simulink model "IDP2_Shehab_Electrical_Systems_Model"  (R2025b)
settings: Solver=VariableStepAuto  StartTime=0.0  StopTime=20  RelTol=1e-3
libraries: nesl_utility x34, fl_lib x32, ee_lib x21, simulink x6
settings Model: Creator=HP VICTUS  LastModifiedBy=HP VICTUS

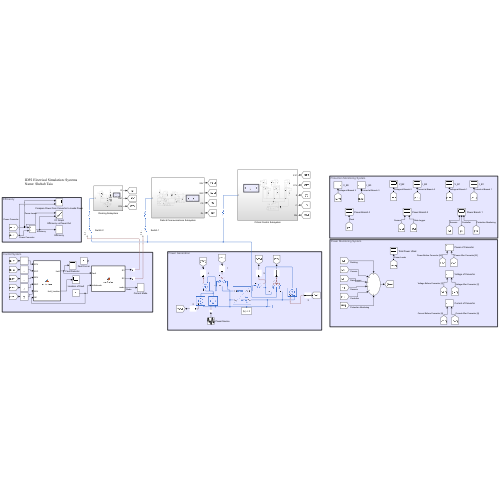
[thumbnail: Simulink's stored preview of the top-level diagram]
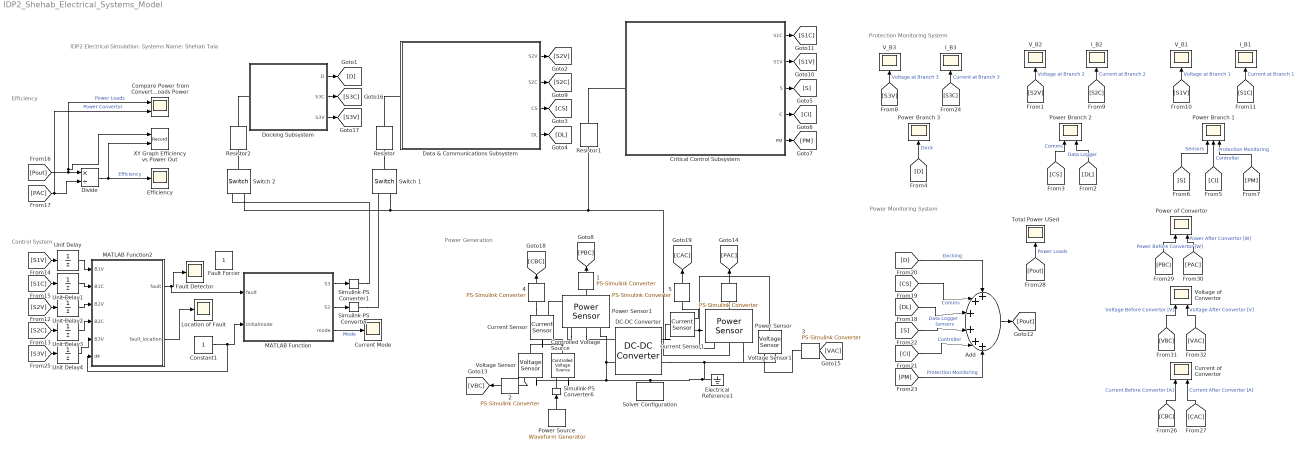
== system IDP2_Shehab_Electrical_Systems_Model ==
  note: Control System
  note: Power Generation
  note: Protection Monitoring System
  note: Power Monitoring System
  note: Efficiency
  note: IDP2 Electrical Simulation: Systems
      | Name: Shehab Taia
   {,1..5} (6 alike) : nesl_utility/PS-Simulink Converter  PhysicalDomain=network_engine_domain  SubClassName=ps_output  LeftPortType=input  RightPortType=output  PseudoPeriodic=off  Frequencies=[]  VectorFormat=1-D array  Unit=1  AffineConversion=off
  Add : Sum  Inputs=++++++
  Compare Power from Convertor to Loads Power : Scope  NumInputPorts=2
      settings: ActiveDisplayYMinimum=79.650776792266242  ActiveDisplayYMaximum=134.0264612610577  DataLoggingVariableName=ScopeData10
  Constant1 : Constant
  Controlled Voltage Source : fl_lib/Electrical/Electrical Sources/Controlled Voltage Source
  Critical Control Subsystem : Subsystem
  Current Mode : Scope
      settings: ActiveDisplayYMinimum=2  ActiveDisplayYMaximum=4  DataLoggingVariableName=ScopeData9
  Current Sensor : fl_lib/Electrical/Electrical Sensors/Current Sensor
  Current Sensor1 : fl_lib/Electrical/Electrical Sensors/Current Sensor
  Current of Convertor : Scope  NumInputPorts=2
      settings: ActiveDisplayYMinimum=0.36664506797171792  ActiveDisplayYMaximum=17.216687272107844  DataLoggingVariableName=ScopeData16
  DC-DC Converter : ee_lib/Semiconductors & Converters/Converters/DC-DC Converter  Vref_option=ee.enum.converters.voltageref.internal  v_ref=24 V  P_rated=250 W  droop_enabled=true  droop_param=ee.enum.converters.droop.value  droop=0.1 V/A  droop_percent=2  Vref_droop=10 V  reversible=ee.enum.converters.directionality.unidirectional  G_diode=1e-8 1/Ohm  P_fixed=2 W  losses_option=ee.enum.converters.lossesOption.proportionalToSquaredCurrent  eff_rated=80  tableOption=ee.enum.converters.lossTableOptionThermal.currentTemp  i_eff_vec=[-2, -1, 1, 2] A  v_eff_vec=[15, 30, 45] V  eff_vec=[66, 76, 80, 74]  eff_2D_table=[66, 66, 66; 76, 76, 76; 80, 80, 80; 74, 74, 74]  model_dynamics=ee.enum.converters.dynamics.yes  tau=0.002 s  v_ini=24 V  v1_min=25 V  R1=1000 Ohm  R2=1000 Ohm  fault_condition=ee.enum.faults.faultInputCondition.greaterThan  fault_threshold=0.5  T_eff_vec=[280, 300, 320] K  eff_3D_table=repmat([66; 76; 80; 74], 1, 3, 3)  thermal_mass=100 J/K  initial_temperature=298.15 K
      settings: InternalSimscapePortConfiguration="{\"Bottom\":[],\"Left\":[{\"id\":\"p1\",\"label\":\"1+\",\"type\":\"foundation.electrical.electrical\"},{\"id\":\"n1\",\"label\":\"1-\",\"type\":\"foundation.electrical.electrical\"}],\"Right\":[{\"id\":\"p2\",\"label\":\"2+\",\"type\":\"foundation.electrical.electrical\"},{\"id\":\"n2\",\"label\":\"2-\",\"type\":\"foundation.electrical.electrical\"}],\"Top\":[]}"
  Data & Communications Subsystem : Subsystem
  Divide : Product  Inputs=*/
  Docking Subsystem : Subsystem
  Efficiency : Scope
      settings: ActiveDisplayYMinimum=0.97227994080182123  ActiveDisplayYMaximum=0.9793482518533968  DataLoggingVariableName=ScopeData11
  Electrical Reference1 : fl_lib/Electrical/Electrical Elements/Electrical Reference
  Fault Detector : Scope
      settings: ActiveDisplayYMinimum=-1.5392337080670928  ActiveDisplayYMaximum=1.140957573182908  DataLoggingVariableName=ScopeData12
  Fault Forcer : Constant
  I_B1 : Scope
      settings: ActiveDisplayYMinimum=2.3119159885086678  ActiveDisplayYMaximum=3.2126875641151642  DataLoggingVariableName=ScopeData8
  I_B2 : Scope
      settings: ActiveDisplayYMinimum=0.94930828791291022  ActiveDisplayYMaximum=2.6489186671968752  DataLoggingVariableName=ScopeData6
  I_B3 : Scope
      settings: ActiveDisplayYMinimum=-1.2813099491745756  ActiveDisplayYMaximum=11.555789758551514  DataLoggingVariableName=ScopeData2
  Location of Fault : Scope
      settings: ActiveDisplayYMinimum=-1  ActiveDisplayYMaximum=1  DataLoggingVariableName=ScopeData3
  MATLAB Function : MATLAB Function  TreatAsAtomicUnit=on
  MATLAB Function2 : MATLAB Function  TreatAsAtomicUnit=on
  Power Branch 1 : Scope  NumInputPorts=3
      settings: ActiveDisplayYMinimum=14.22765652678723  ActiveDisplayYMaximum=23.288334649201424
  Power Branch 2 : Scope  NumInputPorts=2
      settings: ActiveDisplayYMinimum=3.2562727594337782E-13  ActiveDisplayYMaximum=9.0422696415485483E-13
  Power Branch 3 : Scope
      settings: ActiveDisplayYMinimum=-26.0748239794843  ActiveDisplayYMaximum=235.249408902669  DataLoggingVariableName=ScopeData14
  Power Sensor : ee_lib/Sensors & Transducers/Power Sensor  measurement_type=1  averaging_period=1e-4 s
  Power Sensor1 : ee_lib/Sensors & Transducers/Power Sensor  measurement_type=1  averaging_period=1e-4 s
  Power Source : simulink/Sources/Waveform Generator  OutMin=[]  OutMax=[]  OutDataTypeStr=double  SelectedSignal=1  Signals=48 + sin(1, 0.5, 0)  BlockNames=MultiportSwitch_827ba4d7564a4f2  SampleTime=0.1
  Power of Convertor : Scope  NumInputPorts=2
      settings: ActiveDisplayYMinimum=41.30913702815846  ActiveDisplayYMaximum=522.47808402698706  DataLoggingVariableName=ScopeData17
  Resistor : ee_lib/Passive/Resistor  R=0.2 Ohm  enable_R_tol=ee.enum.toleranceApplication.none  R_tol=5  tol_distribution=ee.enum.toleranceDistribution.uniform  nSigma=4  enable_operating_limits=ee.enum.enable.no  operating_limit_action=ee.enum.passive.reportOpLim.warn  power_rating=1 W  max_working_voltage=100 V  noise_mode=ee.enum.sources.noise.Disabled  Tdevice=25 degC  sample_time=1e-3 s  repeatability=ee.enum.ic.repeatability.notRepeatable  user_seed=0  auto_seed=2438775377  power_derating_T1=70 degC  power_derating_T2=155 degC  operating_temperature_range_vec=[-50, 150] degC  alpha=3.93e-3 1/K  Tmeas=25 degC  thermal_mass=100 J/K  temperature_specify=off  temperature_priority=High  temperature=298.15 K  temperature_nominal_specify=off  temperature_nominal_value=1  temperature_nominal_unit=K
  Resistor1 : ee_lib/Passive/Resistor  R=0.2 Ohm  enable_R_tol=ee.enum.toleranceApplication.none  R_tol=5  tol_distribution=ee.enum.toleranceDistribution.uniform  nSigma=4  enable_operating_limits=ee.enum.enable.no  operating_limit_action=ee.enum.passive.reportOpLim.warn  power_rating=1 W  max_working_voltage=100 V  noise_mode=ee.enum.sources.noise.Disabled  Tdevice=25 degC  sample_time=1e-3 s  repeatability=ee.enum.ic.repeatability.notRepeatable  user_seed=0  auto_seed=325791693  power_derating_T1=70 degC  power_derating_T2=155 degC  operating_temperature_range_vec=[-50, 150] degC  alpha=3.93e-3 1/K  Tmeas=25 degC  thermal_mass=100 J/K  temperature_specify=off  temperature_priority=High  temperature=298.15 K  temperature_nominal_specify=off  temperature_nominal_value=1  temperature_nominal_unit=K
  Resistor2 : ee_lib/Passive/Resistor  R=0.2 Ohm  enable_R_tol=ee.enum.toleranceApplication.none  R_tol=5  tol_distribution=ee.enum.toleranceDistribution.uniform  nSigma=4  enable_operating_limits=ee.enum.enable.no  operating_limit_action=ee.enum.passive.reportOpLim.warn  power_rating=1 W  max_working_voltage=100 V  noise_mode=ee.enum.sources.noise.Disabled  Tdevice=25 degC  sample_time=1e-3 s  repeatability=ee.enum.ic.repeatability.notRepeatable  user_seed=0  auto_seed=3807908384  power_derating_T1=70 degC  power_derating_T2=155 degC  operating_temperature_range_vec=[-50, 150] degC  alpha=3.93e-3 1/K  Tmeas=25 degC  thermal_mass=100 J/K  temperature_specify=off  temperature_priority=High  temperature=298.15 K  temperature_nominal_specify=off  temperature_nominal_value=1  temperature_nominal_unit=K
  Simulink-PS Converter : nesl_utility/Simulink-PS Converter  PhysicalDomain=network_engine_domain  SubClassName=ps_input  LeftPortType=input  RightPortType=output  PseudoPeriodic=off  Frequencies=[]  NoiseDistribution=none  NoiseParameters=[]  Unit=1  AffineConversion=off  FilteringAndDerivatives=provide  SimscapeFilterOrder=1  InputFilterTimeConstant=0.001  UdotUserProvided=0
  Simulink-PS Converter1 : nesl_utility/Simulink-PS Converter  PhysicalDomain=network_engine_domain  SubClassName=ps_input  LeftPortType=input  RightPortType=output  PseudoPeriodic=off  Frequencies=[]  NoiseDistribution=none  NoiseParameters=[]  Unit=1  AffineConversion=off  FilteringAndDerivatives=provide  SimscapeFilterOrder=1  InputFilterTimeConstant=0.001  UdotUserProvided=0
  Simulink-PS Converter6 : nesl_utility/Simulink-PS Converter  PhysicalDomain=network_engine_domain  SubClassName=ps_input  LeftPortType=input  RightPortType=output  PseudoPeriodic=off  Frequencies=[]  NoiseDistribution=none  NoiseParameters=[]  Unit=1  AffineConversion=off  FilteringAndDerivatives=filter  SimscapeFilterOrder=1  InputFilterTimeConstant=0.001  UdotUserProvided=0
  Solver Configuration : nesl_utility/Solver Configuration  PhysicalDomain=network_engine_domain  SubClassName=solver  LeftPortType=input  RightPortType=generic  Tones=[]  Harmonics=[]  SimulateNoise=off  Profile=off  UseLocalSampling=off  EnableSwitchedLinearOptims=on  FrequencyDomain=off  UseCCode=off  RelTol=0.001  AbsTol=1e-06  MinStep=1e-09  ToWorkspace=off  RevertToSquareIcSolve=off  NumHomotopyIterations=100  PhasorMode=off  PhasorModeNumHarmonics=1  ConsistencySolver=NEWTON_FTOL  IndexReductionMethod=DerivativeReplacement  DoDC=off  ResidualTolerance=1e-09  ConsistencyTolSource=GLOBAL  ConsistencyAbsTol=0.001  ConsistencyRelTol=0.001  ConsistencyTolFactor=0.001  UseLocalSolver=off  LocalSolverChoice=NE_BACKWARD_EULER_ADVANCER  ResolveIndetEquations=on  FunctionEvalNumThread=1  LocalSolverSampleTime=0.001  DoFixedCost=off  MaxNonlinIter=3  MaxModeIter=2  ComputeImpulses=off  ImpulseIterations=2  LinearAlgebra=Sparse  LinearAlgebraNumThread=0  EquationFormulation=NE_TIME_EF  DelaysMemoryBudget=1024  AutomaticFiltering=on  FilteringTimeConstant=0.001  PartitionStorageMethod=AS_NEEDED  PartitionMemoryBudget=1024  PartitionMethod=FAST  MultibodyUseLocalSolver=off  MultibodyLocalSolverChoice=ODE1  MultibodyLocalSolverSampleTime=0.001
  Switch 1 : fl_lib/Electrical/Electrical Elements/Switch  R_closed=0.01 Ohm  G_open=1e-8 1/Ohm  Threshold=0.5  i_specify=off  i_priority=None  i=0 A  i_nominal_specify=off  i_nominal_value=1  i_nominal_unit=A  v_specify=off  v_priority=None  v=0 V  v_nominal_specify=off  v_nominal_value=1  v_nominal_unit=V
  Switch 2 : fl_lib/Electrical/Electrical Elements/Switch  R_closed=0.01 Ohm  G_open=1e-8 1/Ohm  Threshold=0.5  i_specify=off  i_priority=None  i=0 A  i_nominal_specify=off  i_nominal_value=1  i_nominal_unit=A  v_specify=off  v_priority=None  v=0 V  v_nominal_specify=off  v_nominal_value=1  v_nominal_unit=V
  Total Power USed : Scope
      settings: ActiveDisplayYMinimum=57.08705193849255  ActiveDisplayYMaximum=75.545974460086583  DataLoggingVariableName=ScopeData23
  Unit Delay{,1..4} (5 alike) : UnitDelay  InitialCondition=23  SampleTime=-1  HasFrameUpgradeWarning=on
  V_B1 : Scope
      settings: ActiveDisplayYMinimum=21.641364909946656  ActiveDisplayYMaximum=23.691224490128249  DataLoggingVariableName=ScopeData7
  V_B2 : Scope
      settings: ActiveDisplayYMinimum=21.473361802637658  ActiveDisplayYMaximum=24.098708881242768  DataLoggingVariableName=ScopeData5
  V_B3 : Scope
      settings: ActiveDisplayYMinimum=-0.000306600792252615  ActiveDisplayYMaximum=0.0027003867944249715  DataLoggingVariableName=ScopeData4
  Voltage Sensor : fl_lib/Electrical/Electrical Sensors/Voltage Sensor
  Voltage Sensor1 : fl_lib/Electrical/Electrical Sensors/Voltage Sensor
  Voltage of Convertor : Scope  NumInputPorts=2
      settings: ActiveDisplayYMinimum=19.1344610769676  ActiveDisplayYMaximum=52.318383780373431  DataLoggingVariableName=ScopeData18
  XY Graph Efficiency vs Power Out : Record  NumPorts=2.0  FileSettingsInternal="{\"entries\":[{\"content\":{\"excelSettings\":{\"content\":{},\"type\":\"Streamout.ExcelSettings\"},\"parquetSettings\":{\"content\":{},\"type\":\"Streamout.ParquetSettings\"}},\"type\":\"Streamout.FileSettingStorage\",\"uuid\":\"\"}],\"packageUris\":[\"http:\\/\\/schema.mathworks.com\\/mf0\\/streamout_blocks\\/R2020a\"],\"version\":\"1.0\"}"  FrameSettings=[0, 0]  Layout=[1 1]  SignalsInternal="{\"entries\":[{\"content\":{\"signals\":[{\"content\":{\"blockPath\":[],\"dimensions\":[1],\"domain\":\"\",\"lineColor\":\"#a2142f\",\"plots\":[ 1 ],\"port\":1,\"signalID\":1,\"signalName\":\"Power Loads\"},\"type\":\"RecordBlkView.Signal\",\"uuid\":\"\"},{\"content\":{\"blockPath\":[],\"dimensions\":[1],\"domain\":\"\",\"lineColor\":\"#139fff\",\"plots\":[ 1 ],\"port\":2,\"signalID\":2,\"signalName\":\"Efficiency\"},\"type\":\"RecordBlkView.Signal\",\"uuid\":\"\"}]},\"type\":\"RecordBlkView.InputSignals\",\"uuid\":\"\"}],\"packageUris\":[\"http:\\/\\/schema.mathworks.com\\/mf0\\/streamout_blocks\\/R2020a\"],\"version\":\"1.0\"}"  VisualizationBindings="{\"xyplotplugin\":{\"info\":[{\"series\":[{\"bindingParametersList\":[{\"parameter\":\"X-Axis\",\"signalID\":1,\"signalName\":\"Power Loads\"},{\"parameter\":\"Y-Axis\",\"signalID\":2,\"signalName\":\"Efficiency\"}],\"seriesID\":0}],\"subplotID\":1}]}}"  CompatibilityTag=XY  st=-1
  wires:
  Divide/1 -> XY Graph Efficiency vs Power Out/2, Efficiency/1  "Efficiency"
  [Pout] -> Compare Power from Convertor to Loads Power/1, XY Graph Efficiency vs Power Out/1, Divide/1  "Power Loads"
  [PAC] -> Divide/2, Compare Power from Convertor to Loads Power/2  "Power Convertor"
  MATLAB Function2/2(fault_location) -> Location of Fault/1
  " "/1 -> [PAC]
  Power Source/1 -> Simulink-PS Converter6/1
  Docking Subsystem/1(D) -> [D]
  Data & Communications Subsystem/1(S2V) -> [S2V]
  Data & Communications Subsystem/2(S2C) -> [S2C]
  Data & Communications Subsystem/3(CS) -> [CS]
  Data & Communications Subsystem/4(DL) -> [DL]
  Critical Control Subsystem/1(S1C) -> [S1C]
  Critical Control Subsystem/2(S1V) -> [S1V]
  Critical Control Subsystem/3(S) -> [S]
  Critical Control Subsystem/4(C) -> [CI]
  Critical Control Subsystem/5(PM) -> [PM]
  MATLAB Function/2(S2) -> Simulink-PS Converter/1
  MATLAB Function/1(S3) -> Simulink-PS Converter1/1
  MATLAB Function/3(mode) -> Current Mode/1  "Mode"
  [S2V] -> V_B2/1  "Voltage at Branch 2"
  [S2C] -> I_B2/1  "Current at Branch 2"
  [S1V] -> V_B1/1  "Voltage at Branch 1"
  [S1C] -> I_B1/1  "Current at Branch 1"
  [CS] -> Power Branch 2/1  "Comms"
  [DL] -> Power Branch 2/2  "Data Logger"
  [S] -> Power Branch 1/1  "Sensors"
  [CI] -> Power Branch 1/2  "Controller"
  [PM] -> Power Branch 1/3  "Protection Monitoring"
  [VAC] -> Voltage of Convertor/2  "Voltage After Convertor [V]"
  [VBC] -> Voltage of Convertor/1  "Voltage Before Convertor [V]"
  [PBC] -> Power of Convertor/1  "Power Before Convertor [W]"
  [D] -> Add/1  "Docking"
  [CS] -> Add/2  "Comms"
  [DL] -> Add/3  "Data Logger"
  [S] -> Add/4  "Sensors"
  [CI] -> Add/5  "Controller"
  [PM] -> Add/6  "Protection Monitoring"
  Add/1 -> [Pout]
  " 3"/1 -> [VAC]
  [PAC] -> Power of Convertor/2  "Power After Convertor [W]"
  " 2"/1 -> [VBC]
  Docking Subsystem/2(S3C) -> [S3C]
  Docking Subsystem/3(S3V) -> [S3V]
  [S3C] -> I_B3/1  "Current at Branch 3"
  [S3V] -> V_B3/1  "Voltage at Branch 3"
  [S1V] -> Unit Delay/1
  [S2C] -> Unit Delay3/1
  [S1C] -> Unit Delay1/1
  [S2V] -> Unit Delay2/1
  [S3V] -> Unit Delay4/1
  Unit Delay3/1 -> MATLAB Function2/4(B2C)
  Unit Delay2/1 -> MATLAB Function2/3(B2V)
  Unit Delay1/1 -> MATLAB Function2/2(B1C)
  Unit Delay/1 -> MATLAB Function2/1(B1V)
  Unit Delay4/1 -> MATLAB Function2/5(B3V)
  Constant1/1 -> MATLAB Function2/6(IM), MATLAB Function/2(initialmode)
  MATLAB Function2/1(fault) -> MATLAB Function/1(fault), Fault Detector/1
  " 4"/1 -> [CBC]
  " 5"/1 -> [CAC]
  [CBC] -> Current of Convertor/1  "Current Before Convertor [A]"
  [CAC] -> Current of Convertor/2  "Current After Convertor [A]"
  " 1"/1 -> [PBC]
  [D] -> Power Branch 3/1  "Dock"
  [Pout] -> Total Power USed/1  "Power Loads"
  connections:
  Power Sensor1/LConn1 -- Current Sensor/RConn2
  Simulink-PS Converter6/RConn1 -- Controlled Voltage Source/RConn1
  Resistor/LConn1 -- Switch 1/LConn1
  Switch 1/RConn2 -- Power Sensor/LConn2 -- Resistor1/LConn1 -- Switch 2/RConn2
  Switch 2/LConn1 -- Resistor2/LConn1
  Resistor/RConn1 -- Data & Communications Subsystem/LConn1
  DC-DC Converter/RConn2 -- Power Sensor/LConn3 -- Voltage Sensor1/RConn2 -- Solver Configuration/RConn1 -- Voltage Sensor/RConn2 -- Controlled Voltage Source/RConn2 -- Power Sensor1/LConn3 -- DC-DC Converter/LConn2 -- Electrical Reference1/LConn1
  Critical Control Subsystem/LConn1 -- Resistor1/RConn1
  Voltage Sensor1/LConn1 -- Power Sensor/LConn1 -- Current Sensor1/RConn2
  " "/LConn1 -- Power Sensor/RConn1
  Power Sensor1/RConn1 -- " 1"/LConn1
  " 2"/LConn1 -- Voltage Sensor/RConn1
  " 3"/LConn1 -- Voltage Sensor1/RConn1
  Power Sensor1/LConn2 -- DC-DC Converter/LConn1
  Simulink-PS Converter1/RConn1 -- Switch 2/RConn1
  Simulink-PS Converter/RConn1 -- Switch 1/RConn1
  Resistor2/RConn1 -- Docking Subsystem/LConn1
  Current Sensor/LConn1 -- Controlled Voltage Source/LConn1 -- Voltage Sensor/LConn1
  " 4"/LConn1 -- Current Sensor/RConn1
  DC-DC Converter/RConn1 -- Current Sensor1/LConn1
  " 5"/LConn1 -- Current Sensor1/RConn1

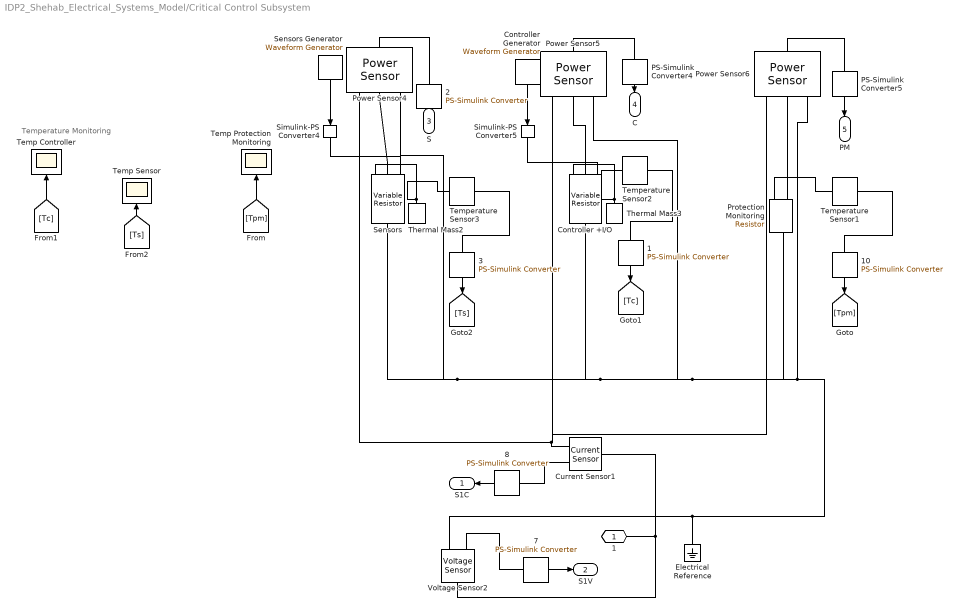
== system IDP2_Shehab_Electrical_Systems_Model/Critical Control Subsystem ==
  note: Temperature Monitoring
   {1..3,7..8,10} (6 alike) : nesl_utility/PS-Simulink Converter  PhysicalDomain=network_engine_domain  SubClassName=ps_output  LeftPortType=input  RightPortType=output  PseudoPeriodic=off  Frequencies=[]  VectorFormat=1-D array  Unit=1  AffineConversion=off
  Controller Generator : simulink/Sources/Waveform Generator  OutMin=[]  OutMax=[]  OutDataTypeStr=double  SelectedSignal=1  Signals=step(5, 23.04, 16.46) + step(6, 0, 6.58)  BlockNames=MultiportSwitch_3dca4f294659435  SampleTime=0.1
  Controller +I/O : fl_lib/Electrical/Electrical Elements/Variable Resistor  Rmin=0 Ohm  thermalEnable=true  thermal_mass=0 J/K  i_specify=off  i_priority=None  i=0 A  i_nominal_specify=off  i_nominal_value=1  i_nominal_unit=A  v_specify=off  v_priority=None  v=0 V  v_nominal_specify=off  v_nominal_value=1  v_nominal_unit=V  T_specify=off  T_priority=None  T=300 K  T_nominal_specify=off  T_nominal_value=1  T_nominal_unit=K
      settings: InternalSimscapePortConfiguration="{\"Bottom\":[],\"Left\":[{\"id\":\"R\",\"label\":\"R\",\"type\":\"input\"},{\"id\":\"p\",\"label\":\"+\",\"type\":\"foundation.electrical.electrical\"}],\"Right\":[{\"id\":\"n\",\"label\":\"-\",\"type\":\"foundation.electrical.electrical\"}],\"Top\":[{\"id\":\"H\",\"label\":\"H\",\"type\":\"foundation.thermal.thermal\"}]}"
  Current Sensor1 : fl_lib/Electrical/Electrical Sensors/Current Sensor
  Electrical Reference : fl_lib/Electrical/Electrical Elements/Electrical Reference
  PS-Simulink Converter4 : nesl_utility/PS-Simulink Converter  PhysicalDomain=network_engine_domain  SubClassName=ps_output  LeftPortType=input  RightPortType=output  PseudoPeriodic=off  Frequencies=[]  VectorFormat=1-D array  Unit=1  AffineConversion=off
  PS-Simulink Converter5 : nesl_utility/PS-Simulink Converter  PhysicalDomain=network_engine_domain  SubClassName=ps_output  LeftPortType=input  RightPortType=output  PseudoPeriodic=off  Frequencies=[]  VectorFormat=1-D array  Unit=1  AffineConversion=off
  Power Sensor4 : ee_lib/Sensors & Transducers/Power Sensor  measurement_type=1  averaging_period=1e-4 s
  Power Sensor5 : ee_lib/Sensors & Transducers/Power Sensor  measurement_type=1  averaging_period=1e-4 s
  Power Sensor6 : ee_lib/Sensors & Transducers/Power Sensor  measurement_type=1  averaging_period=1e-4 s
  Protection Monitoring : ee_lib/Passive/Resistor  R=28.8 Ohm  enable_R_tol=ee.enum.toleranceApplication.none  R_tol=5  tol_distribution=ee.enum.toleranceDistribution.uniform  nSigma=4  enable_operating_limits=ee.enum.enable.no  operating_limit_action=ee.enum.passive.reportOpLim.warn  power_rating=1 W  max_working_voltage=100 V  noise_mode=ee.enum.sources.noise.Disabled  Tdevice=25 degC  sample_time=1e-3 s  repeatability=ee.enum.ic.repeatability.notRepeatable  user_seed=0  auto_seed=1119815447  power_derating_T1=70 degC  power_derating_T2=155 degC  operating_temperature_range_vec=[-50, 150] degC  alpha=3.93e-3 1/K  Tmeas=25 degC  thermal_mass=200 J/K  temperature_specify=off  temperature_priority=High  temperature=298.15 K  temperature_nominal_specify=off  temperature_nominal_value=1  temperature_nominal_unit=K
      settings: InternalSimscapePortConfiguration="{\"Bottom\":[],\"Left\":[{\"id\":\"p\",\"label\":\"+\",\"type\":\"foundation.electrical.electrical\"},{\"id\":\"H\",\"label\":\"H\",\"type\":\"foundation.thermal.thermal\"}],\"Right\":[{\"id\":\"n\",\"label\":\"-\",\"type\":\"foundation.electrical.electrical\"}],\"Top\":[]}"
  Sensors : fl_lib/Electrical/Electrical Elements/Variable Resistor  Rmin=0 Ohm  thermalEnable=true  thermal_mass=0 J/K  i_specify=off  i_priority=None  i=0 A  i_nominal_specify=off  i_nominal_value=1  i_nominal_unit=A  v_specify=off  v_priority=None  v=0 V  v_nominal_specify=off  v_nominal_value=1  v_nominal_unit=V  T_specify=off  T_priority=None  T=300 K  T_nominal_specify=off  T_nominal_value=1  T_nominal_unit=K
      settings: InternalSimscapePortConfiguration="{\"Bottom\":[],\"Left\":[{\"id\":\"R\",\"label\":\"R\",\"type\":\"input\"},{\"id\":\"p\",\"label\":\"+\",\"type\":\"foundation.electrical.electrical\"}],\"Right\":[{\"id\":\"n\",\"label\":\"-\",\"type\":\"foundation.electrical.electrical\"}],\"Top\":[{\"id\":\"H\",\"label\":\"H\",\"type\":\"foundation.thermal.thermal\"}]}"
  Sensors Generator : simulink/Sources/Waveform Generator  OutMin=[]  OutMax=[]  OutDataTypeStr=double  SelectedSignal=1  Signals=step(3, 32, 23.04) + step(10, 0, 32-23.04)  BlockNames=MultiportSwitch_565f76e57e2d47f  SampleTime=0.1
  Simulink-PS Converter4 : nesl_utility/Simulink-PS Converter  PhysicalDomain=network_engine_domain  SubClassName=ps_input  LeftPortType=input  RightPortType=output  PseudoPeriodic=off  Frequencies=[]  NoiseDistribution=none  NoiseParameters=[]  Unit=1  AffineConversion=off  FilteringAndDerivatives=filter  SimscapeFilterOrder=1  InputFilterTimeConstant=0.001  UdotUserProvided=0
  Simulink-PS Converter5 : nesl_utility/Simulink-PS Converter  PhysicalDomain=network_engine_domain  SubClassName=ps_input  LeftPortType=input  RightPortType=output  PseudoPeriodic=off  Frequencies=[]  NoiseDistribution=none  NoiseParameters=[]  Unit=1  AffineConversion=off  FilteringAndDerivatives=filter  SimscapeFilterOrder=1  InputFilterTimeConstant=0.001  UdotUserProvided=0
  Temp Controller : Scope
      settings: ActiveDisplayYMinimum=292.94814557194843  ActiveDisplayYMaximum=294.96668985246413  DataLoggingVariableName=ScopeData19
  Temp Protection Monitoring : Scope
      settings: ActiveDisplayYMinimum=297.9369765879818  ActiveDisplayYMaximum=300.06721070816349  DataLoggingVariableName=ScopeData13
  Temp Sensor : Scope
      settings: ActiveDisplayYMinimum=292.66432897393719  ActiveDisplayYMaximum=297.52103923456542  DataLoggingVariableName=ScopeData20
  Temperature Sensor1 : fl_lib/Thermal/Thermal Sensors/Temperature Sensor  temperature_measure=foundation.enum.MeasurementReference.absolute
      settings: InternalSimscapePortConfiguration="{\"Bottom\":[],\"Left\":[{\"id\":\"A\",\"label\":\"A\",\"type\":\"foundation.thermal.thermal\"}],\"Right\":[{\"id\":\"T\",\"label\":\"T\",\"type\":\"output\"}],\"Top\":[]}"
  Temperature Sensor2 : fl_lib/Thermal/Thermal Sensors/Temperature Sensor  temperature_measure=foundation.enum.MeasurementReference.absolute
      settings: InternalSimscapePortConfiguration="{\"Bottom\":[],\"Left\":[{\"id\":\"A\",\"label\":\"A\",\"type\":\"foundation.thermal.thermal\"}],\"Right\":[{\"id\":\"T\",\"label\":\"T\",\"type\":\"output\"}],\"Top\":[]}"
  Temperature Sensor3 : fl_lib/Thermal/Thermal Sensors/Temperature Sensor  temperature_measure=foundation.enum.MeasurementReference.absolute
      settings: InternalSimscapePortConfiguration="{\"Bottom\":[],\"Left\":[{\"id\":\"A\",\"label\":\"A\",\"type\":\"foundation.thermal.thermal\"}],\"Right\":[{\"id\":\"T\",\"label\":\"T\",\"type\":\"output\"}],\"Top\":[]}"
  Thermal Mass2 : fl_lib/Thermal/Thermal Elements/Thermal Mass  mass_type=foundation.enum.constant_variable.constant  mass=1 kg  sp_heat=90 J/(K*kg)  mass_min=1e-6 kg  num_ports=foundation.enum.numPorts2.one  m_specify=off  m_priority=High  m=1 kg  m_nominal_specify=off  m_nominal_value=1  m_nominal_unit=kg  T_specify=on  T_priority=Low  T=293.15 K  T_nominal_specify=off  T_nominal_value=1  T_nominal_unit=K  Q_specify=off  Q_priority=None  Q=0 W  Q_nominal_specify=off  Q_nominal_value=1  Q_nominal_unit=W
  Thermal Mass3 : fl_lib/Thermal/Thermal Elements/Thermal Mass  mass_type=foundation.enum.constant_variable.constant  mass=1 kg  sp_heat=270 J/(K*kg)  mass_min=1e-6 kg  num_ports=foundation.enum.numPorts2.one  m_specify=off  m_priority=High  m=1 kg  m_nominal_specify=off  m_nominal_value=1  m_nominal_unit=kg  T_specify=on  T_priority=Low  T=293.15 K  T_nominal_specify=off  T_nominal_value=1  T_nominal_unit=K  Q_specify=off  Q_priority=None  Q=0 W  Q_nominal_specify=off  Q_nominal_value=1  Q_nominal_unit=W
  Voltage Sensor2 : fl_lib/Electrical/Electrical Sensors/Voltage Sensor
  1 : PMIOPort  Side=Left
  S1C : Outport
  S1V : Outport  Port=2
  S : Outport  Port=3
  C : Outport  Port=4
  PM : Outport  Port=5
  wires:
  Controller Generator/1 -> Simulink-PS Converter5/1
  Sensors Generator/1 -> Simulink-PS Converter4/1
  " 2"/1 -> S/1
  " 8"/1 -> S1C/1
  " 7"/1 -> S1V/1
  PS-Simulink Converter4/1 -> C/1
  PS-Simulink Converter5/1 -> PM/1
  " 10"/1 -> [Tpm]
  [Tpm] -> Temp Protection Monitoring/1
  [Tc] -> Temp Controller/1
  [Ts] -> Temp Sensor/1
  " 1"/1 -> [Tc]
  " 3"/1 -> [Ts]
  connections:
  Power Sensor6/LConn3 -- Protection Monitoring/RConn1 -- Power Sensor5/LConn3 -- Controller +I/O/RConn1 -- Power Sensor4/LConn3 -- Sensors/RConn1 -- Voltage Sensor2/RConn2 -- Electrical Reference/LConn1
  Current Sensor1/RConn1 -- " 8"/LConn1
  Temperature Sensor1/LConn1 -- Protection Monitoring/LConn2
  Power Sensor6/LConn2 -- Protection Monitoring/LConn1
  Thermal Mass3/LConn1 -- Temperature Sensor2/LConn1 -- Controller +I/O/LConn3
  PS-Simulink Converter4/LConn1 -- Power Sensor5/RConn1
  " 10"/LConn1 -- Temperature Sensor1/RConn1
  Current Sensor1/LConn1 -- Voltage Sensor2/LConn1 -- 1/RConn1
  PS-Simulink Converter5/LConn1 -- Power Sensor6/RConn1
  Thermal Mass2/LConn1 -- Temperature Sensor3/LConn1 -- Sensors/LConn3
  Current Sensor1/RConn2 -- Power Sensor6/LConn1 -- Power Sensor5/LConn1 -- Power Sensor4/LConn1
  Power Sensor5/LConn2 -- Controller +I/O/LConn2
  Controller +I/O/LConn1 -- Simulink-PS Converter5/RConn1
  " 2"/LConn1 -- Power Sensor4/RConn1
  Simulink-PS Converter4/RConn1 -- Sensors/LConn1
  Voltage Sensor2/RConn1 -- " 7"/LConn1
  Sensors/LConn2 -- Power Sensor4/LConn2
  " 1"/LConn1 -- Temperature Sensor2/RConn1
  " 3"/LConn1 -- Temperature Sensor3/RConn1

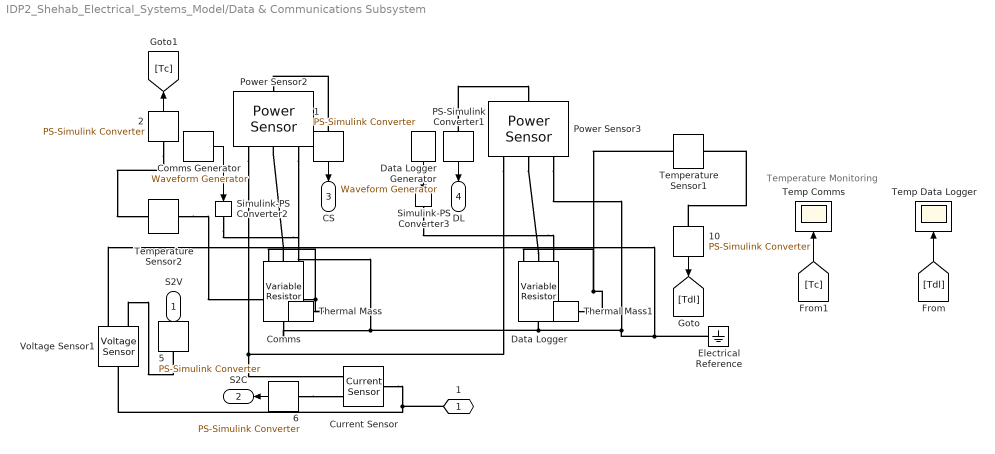
== system IDP2_Shehab_Electrical_Systems_Model/Data & Communications Subsystem ==
  note: Temperature Monitoring
   {1..2,5..6,10} (5 alike) : nesl_utility/PS-Simulink Converter  PhysicalDomain=network_engine_domain  SubClassName=ps_output  LeftPortType=input  RightPortType=output  PseudoPeriodic=off  Frequencies=[]  VectorFormat=1-D array  Unit=1  AffineConversion=off
  Comms : fl_lib/Electrical/Electrical Elements/Variable Resistor  Rmin=0 Ohm  thermalEnable=true  thermal_mass=0 J/K  i_specify=off  i_priority=None  i=0 A  i_nominal_specify=off  i_nominal_value=1  i_nominal_unit=A  v_specify=off  v_priority=None  v=0 V  v_nominal_specify=off  v_nominal_value=1  v_nominal_unit=V  T_specify=off  T_priority=None  T=300 K  T_nominal_specify=off  T_nominal_value=1  T_nominal_unit=K
      settings: InternalSimscapePortConfiguration="{\"Bottom\":[],\"Left\":[{\"id\":\"R\",\"label\":\"R\",\"type\":\"input\"},{\"id\":\"p\",\"label\":\"+\",\"type\":\"foundation.electrical.electrical\"}],\"Right\":[{\"id\":\"n\",\"label\":\"-\",\"type\":\"foundation.electrical.electrical\"}],\"Top\":[{\"id\":\"H\",\"label\":\"H\",\"type\":\"foundation.thermal.thermal\"}]}"
  Comms Generator : simulink/Sources/Waveform Generator  OutMin=[]  OutMax=[]  OutDataTypeStr=double  SelectedSignal=1  Signals=step(5, 28.8, 11.52)  BlockNames=MultiportSwitch_095543f3cf194af  SampleTime=0.1
  Current Sensor : fl_lib/Electrical/Electrical Sensors/Current Sensor
  Data Logger : fl_lib/Electrical/Electrical Elements/Variable Resistor  Rmin=0 Ohm  thermalEnable=true  thermal_mass=0 J/K  i_specify=off  i_priority=None  i=0 A  i_nominal_specify=off  i_nominal_value=1  i_nominal_unit=A  v_specify=off  v_priority=None  v=0 V  v_nominal_specify=off  v_nominal_value=1  v_nominal_unit=V  T_specify=off  T_priority=None  T=300 K  T_nominal_specify=off  T_nominal_value=1  T_nominal_unit=K
      settings: InternalSimscapePortConfiguration="{\"Bottom\":[],\"Left\":[{\"id\":\"R\",\"label\":\"R\",\"type\":\"input\"},{\"id\":\"p\",\"label\":\"+\",\"type\":\"foundation.electrical.electrical\"}],\"Right\":[{\"id\":\"n\",\"label\":\"-\",\"type\":\"foundation.electrical.electrical\"}],\"Top\":[{\"id\":\"H\",\"label\":\"H\",\"type\":\"foundation.thermal.thermal\"}]}"
  Data Logger Generator : simulink/Sources/Waveform Generator  OutMin=[]  OutMax=[]  OutDataTypeStr=double  SelectedSignal=1  Signals=step(7, 72, 38.4)  BlockNames=MultiportSwitch_7b4fce7a58b2408  SampleTime=0.1
  Electrical Reference : fl_lib/Electrical/Electrical Elements/Electrical Reference
  PS-Simulink Converter1 : nesl_utility/PS-Simulink Converter  PhysicalDomain=network_engine_domain  SubClassName=ps_output  LeftPortType=input  RightPortType=output  PseudoPeriodic=off  Frequencies=[]  VectorFormat=1-D array  Unit=1  AffineConversion=off
  Power Sensor2 : ee_lib/Sensors & Transducers/Power Sensor  measurement_type=1  averaging_period=1e-4 s
  Power Sensor3 : ee_lib/Sensors & Transducers/Power Sensor  measurement_type=1  averaging_period=1e-4 s
  Simulink-PS Converter2 : nesl_utility/Simulink-PS Converter  PhysicalDomain=network_engine_domain  SubClassName=ps_input  LeftPortType=input  RightPortType=output  PseudoPeriodic=off  Frequencies=[]  NoiseDistribution=none  NoiseParameters=[]  Unit=1  AffineConversion=off  FilteringAndDerivatives=filter  SimscapeFilterOrder=1  InputFilterTimeConstant=0.001  UdotUserProvided=0
  Simulink-PS Converter3 : nesl_utility/Simulink-PS Converter  PhysicalDomain=network_engine_domain  SubClassName=ps_input  LeftPortType=input  RightPortType=output  PseudoPeriodic=off  Frequencies=[]  NoiseDistribution=none  NoiseParameters=[]  Unit=1  AffineConversion=off  FilteringAndDerivatives=filter  SimscapeFilterOrder=1  InputFilterTimeConstant=0.001  UdotUserProvided=0
  Temp Comms : Scope
      settings: ActiveDisplayYMinimum=292.94814557194843  ActiveDisplayYMaximum=294.96668985246413  DataLoggingVariableName=ScopeData21
  "Temp Data Logger " : Scope
      settings: ActiveDisplayYMinimum=293.00152884444793  ActiveDisplayYMaximum=294.48624039996855  DataLoggingVariableName=ScopeData22
  Temperature Sensor1 : fl_lib/Thermal/Thermal Sensors/Temperature Sensor  temperature_measure=foundation.enum.MeasurementReference.absolute
      settings: InternalSimscapePortConfiguration="{\"Bottom\":[],\"Left\":[{\"id\":\"A\",\"label\":\"A\",\"type\":\"foundation.thermal.thermal\"}],\"Right\":[{\"id\":\"T\",\"label\":\"T\",\"type\":\"output\"}],\"Top\":[]}"
  Temperature Sensor2 : fl_lib/Thermal/Thermal Sensors/Temperature Sensor  temperature_measure=foundation.enum.MeasurementReference.absolute
      settings: InternalSimscapePortConfiguration="{\"Bottom\":[],\"Left\":[{\"id\":\"A\",\"label\":\"A\",\"type\":\"foundation.thermal.thermal\"}],\"Right\":[{\"id\":\"T\",\"label\":\"T\",\"type\":\"output\"}],\"Top\":[]}"
  Thermal Mass : fl_lib/Thermal/Thermal Elements/Thermal Mass  mass_type=foundation.enum.constant_variable.constant  mass=1 kg  sp_heat="500  J/(K*kg)"  mass_min=1e-6 kg  num_ports=foundation.enum.numPorts2.one  m_specify=off  m_priority=High  m=1 kg  m_nominal_specify=off  m_nominal_value=1  m_nominal_unit=kg  T_specify=on  T_priority=Low  T=293.15 K  T_nominal_specify=off  T_nominal_value=1  T_nominal_unit=K  Q_specify=off  Q_priority=None  Q=0 W  Q_nominal_specify=off  Q_nominal_value=1  Q_nominal_unit=W
  Thermal Mass1 : fl_lib/Thermal/Thermal Elements/Thermal Mass  mass_type=foundation.enum.constant_variable.constant  mass=1 kg  sp_heat=180 J/(K*kg)  mass_min=1e-6 kg  num_ports=foundation.enum.numPorts2.one  m_specify=off  m_priority=High  m=1 kg  m_nominal_specify=off  m_nominal_value=1  m_nominal_unit=kg  T_specify=on  T_priority=Low  T=293.15 K  T_nominal_specify=off  T_nominal_value=1  T_nominal_unit=K  Q_specify=off  Q_priority=None  Q=0 W  Q_nominal_specify=off  Q_nominal_value=1  Q_nominal_unit=W
  Voltage Sensor1 : fl_lib/Electrical/Electrical Sensors/Voltage Sensor
  1 : PMIOPort  Side=Left
  S2V : Outport
  S2C : Outport  Port=2
  CS : Outport  Port=3
  DL : Outport  Port=4
  wires:
  Comms Generator/1 -> Simulink-PS Converter2/1
  Data Logger Generator/1 -> Simulink-PS Converter3/1
  " 5"/1 -> S2V/1
  " 6"/1 -> S2C/1
  " 1"/1 -> CS/1
  PS-Simulink Converter1/1 -> DL/1
  [Tc] -> Temp Comms/1
  [Tdl] -> "Temp Data Logger "/1
  " 10"/1 -> [Tdl]
  " 2"/1 -> [Tc]
  connections:
  Voltage Sensor1/RConn2 -- Comms/RConn1 -- Power Sensor2/LConn3 -- Data Logger/RConn1 -- Power Sensor3/LConn3 -- Electrical Reference/LConn1
  Current Sensor/LConn1 -- Voltage Sensor1/LConn1 -- 1/RConn1
  " 1"/LConn1 -- Power Sensor2/RConn1
  Thermal Mass/LConn1 -- Temperature Sensor2/LConn1 -- Comms/LConn3
  Power Sensor2/LConn1 -- Power Sensor3/LConn1 -- Current Sensor/RConn2
  Comms/LConn2 -- Power Sensor2/LConn2
  " 6"/LConn1 -- Current Sensor/RConn1
  PS-Simulink Converter1/LConn1 -- Power Sensor3/RConn1
  Simulink-PS Converter2/RConn1 -- Comms/LConn1
  Power Sensor3/LConn2 -- Data Logger/LConn2
  Thermal Mass1/LConn1 -- Temperature Sensor1/LConn1 -- Data Logger/LConn3
  Simulink-PS Converter3/RConn1 -- Data Logger/LConn1
  Voltage Sensor1/RConn1 -- " 5"/LConn1
  " 10"/LConn1 -- Temperature Sensor1/RConn1
  " 2"/LConn1 -- Temperature Sensor2/RConn1

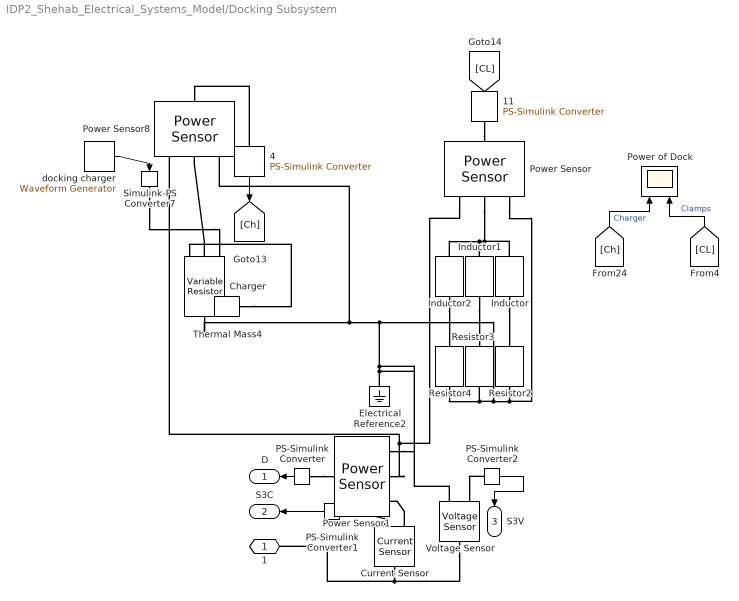
== system IDP2_Shehab_Electrical_Systems_Model/Docking Subsystem ==
  " 11" : nesl_utility/PS-Simulink Converter  PhysicalDomain=network_engine_domain  SubClassName=ps_output  LeftPortType=input  RightPortType=output  PseudoPeriodic=off  Frequencies=[]  VectorFormat=1-D array  Unit=1  AffineConversion=off
  " 4" : nesl_utility/PS-Simulink Converter  PhysicalDomain=network_engine_domain  SubClassName=ps_output  LeftPortType=input  RightPortType=output  PseudoPeriodic=off  Frequencies=[]  VectorFormat=1-D array  Unit=1  AffineConversion=off
  Charger : fl_lib/Electrical/Electrical Elements/Variable Resistor  Rmin=0 Ohm  thermalEnable=true  thermal_mass=0 J/K  i_specify=off  i_priority=None  i=0 A  i_nominal_specify=off  i_nominal_value=1  i_nominal_unit=A  v_specify=off  v_priority=None  v=0 V  v_nominal_specify=off  v_nominal_value=1  v_nominal_unit=V  T_specify=off  T_priority=None  T=300 K  T_nominal_specify=off  T_nominal_value=1  T_nominal_unit=K
      settings: InternalSimscapePortConfiguration="{\"Bottom\":[],\"Left\":[{\"id\":\"R\",\"label\":\"R\",\"type\":\"input\"},{\"id\":\"p\",\"label\":\"+\",\"type\":\"foundation.electrical.electrical\"}],\"Right\":[{\"id\":\"n\",\"label\":\"-\",\"type\":\"foundation.electrical.electrical\"}],\"Top\":[{\"id\":\"H\",\"label\":\"H\",\"type\":\"foundation.thermal.thermal\"}]}"
  Current Sensor : fl_lib/Electrical/Electrical Sensors/Current Sensor
  Electrical Reference2 : fl_lib/Electrical/Electrical Elements/Electrical Reference
  Inductor : ee_lib/Passive/Inductor  l=50 mH  enable_L_tol=ee.enum.toleranceApplication.none  L_tol=20  tol_distribution=ee.enum.toleranceDistribution.uniform  nSigma=4  r=0 Ohm  g=1e-9 1/Ohm  enable_operating_limits=ee.enum.enable.no  operating_limit_action=ee.enum.passive.reportOpLim.warn  max_working_current=1 A  power_rating=1 W  i_L_specify=off  i_L_priority=High  i_L=0 A  i_L_nominal_specify=off  i_L_nominal_value=1  i_L_nominal_unit=A
  Inductor1 : ee_lib/Passive/Inductor  l=50 mH  enable_L_tol=ee.enum.toleranceApplication.none  L_tol=20  tol_distribution=ee.enum.toleranceDistribution.uniform  nSigma=4  r=0 Ohm  g=1e-9 1/Ohm  enable_operating_limits=ee.enum.enable.no  operating_limit_action=ee.enum.passive.reportOpLim.warn  max_working_current=1 A  power_rating=1 W  i_L_specify=off  i_L_priority=High  i_L=0 A  i_L_nominal_specify=off  i_L_nominal_value=1  i_L_nominal_unit=A
  Inductor2 : ee_lib/Passive/Inductor  l=50 mH  enable_L_tol=ee.enum.toleranceApplication.none  L_tol=20  tol_distribution=ee.enum.toleranceDistribution.uniform  nSigma=4  r=0 Ohm  g=1e-9 1/Ohm  enable_operating_limits=ee.enum.enable.no  operating_limit_action=ee.enum.passive.reportOpLim.warn  max_working_current=1 A  power_rating=1 W  i_L_specify=off  i_L_priority=High  i_L=0 A  i_L_nominal_specify=off  i_L_nominal_value=1  i_L_nominal_unit=A
  PS-Simulink Converter : nesl_utility/PS-Simulink Converter  PhysicalDomain=network_engine_domain  SubClassName=ps_output  LeftPortType=input  RightPortType=output  PseudoPeriodic=off  Frequencies=[]  VectorFormat=inherit  Unit=inherit  AffineConversion=off
  PS-Simulink Converter1 : nesl_utility/PS-Simulink Converter  PhysicalDomain=network_engine_domain  SubClassName=ps_output  LeftPortType=input  RightPortType=output  PseudoPeriodic=off  Frequencies=[]  VectorFormat=inherit  Unit=inherit  AffineConversion=off
  PS-Simulink Converter2 : nesl_utility/PS-Simulink Converter  PhysicalDomain=network_engine_domain  SubClassName=ps_output  LeftPortType=input  RightPortType=output  PseudoPeriodic=off  Frequencies=[]  VectorFormat=inherit  Unit=inherit  AffineConversion=off
  Power Sensor : ee_lib/Sensors & Transducers/Power Sensor  measurement_type=1  averaging_period=1e-4 s
  Power Sensor1 : ee_lib/Sensors & Transducers/Power Sensor  measurement_type=1  averaging_period=1e-4 s
  Power Sensor8 : ee_lib/Sensors & Transducers/Power Sensor  measurement_type=1  averaging_period=1e-4 s
  Power of Dock : Scope  NumInputPorts=2
      settings: ActiveDisplayYMinimum=-21.485356525822223  ActiveDisplayYMaximum=193.90012449610464  DataLoggingVariableName=ScopeData15
  Resistor2 : ee_lib/Passive/Resistor  R=19.2 Ohm  enable_R_tol=ee.enum.toleranceApplication.none  R_tol=5  tol_distribution=ee.enum.toleranceDistribution.uniform  nSigma=4  enable_operating_limits=ee.enum.enable.no  operating_limit_action=ee.enum.passive.reportOpLim.warn  power_rating=1 W  max_working_voltage=100 V  noise_mode=ee.enum.sources.noise.Disabled  Tdevice=25 degC  sample_time=1e-3 s  repeatability=ee.enum.ic.repeatability.notRepeatable  user_seed=0  auto_seed=546603451  power_derating_T1=70 degC  power_derating_T2=155 degC  operating_temperature_range_vec=[-50, 150] degC  alpha=3.93e-3 1/K  Tmeas=25 degC  thermal_mass=100 J/K  temperature_specify=off  temperature_priority=High  temperature=298.15 K  temperature_nominal_specify=off  temperature_nominal_value=1  temperature_nominal_unit=K
  Resistor3 : ee_lib/Passive/Resistor  R=19.2 Ohm  enable_R_tol=ee.enum.toleranceApplication.none  R_tol=5  tol_distribution=ee.enum.toleranceDistribution.uniform  nSigma=4  enable_operating_limits=ee.enum.enable.no  operating_limit_action=ee.enum.passive.reportOpLim.warn  power_rating=1 W  max_working_voltage=100 V  noise_mode=ee.enum.sources.noise.Disabled  Tdevice=25 degC  sample_time=1e-3 s  repeatability=ee.enum.ic.repeatability.notRepeatable  user_seed=0  auto_seed=37141537  power_derating_T1=70 degC  power_derating_T2=155 degC  operating_temperature_range_vec=[-50, 150] degC  alpha=3.93e-3 1/K  Tmeas=25 degC  thermal_mass=100 J/K  temperature_specify=off  temperature_priority=High  temperature=298.15 K  temperature_nominal_specify=off  temperature_nominal_value=1  temperature_nominal_unit=K
  Resistor4 : ee_lib/Passive/Resistor  R=19.2 Ohm  enable_R_tol=ee.enum.toleranceApplication.none  R_tol=5  tol_distribution=ee.enum.toleranceDistribution.uniform  nSigma=4  enable_operating_limits=ee.enum.enable.no  operating_limit_action=ee.enum.passive.reportOpLim.warn  power_rating=1 W  max_working_voltage=100 V  noise_mode=ee.enum.sources.noise.Disabled  Tdevice=25 degC  sample_time=1e-3 s  repeatability=ee.enum.ic.repeatability.notRepeatable  user_seed=0  auto_seed=3122783108  power_derating_T1=70 degC  power_derating_T2=155 degC  operating_temperature_range_vec=[-50, 150] degC  alpha=3.93e-3 1/K  Tmeas=25 degC  thermal_mass=100 J/K  temperature_specify=off  temperature_priority=High  temperature=298.15 K  temperature_nominal_specify=off  temperature_nominal_value=1  temperature_nominal_unit=K
  Simulink-PS Converter7 : nesl_utility/Simulink-PS Converter  PhysicalDomain=network_engine_domain  SubClassName=ps_input  LeftPortType=input  RightPortType=output  PseudoPeriodic=off  Frequencies=[]  NoiseDistribution=none  NoiseParameters=[]  Unit=1  AffineConversion=off  FilteringAndDerivatives=filter  SimscapeFilterOrder=1  InputFilterTimeConstant=0.001  UdotUserProvided=0
  Thermal Mass4 : fl_lib/Thermal/Thermal Elements/Thermal Mass  mass_type=foundation.enum.constant_variable.constant  mass=2 kg  sp_heat=900 J/(K*kg)  mass_min=1e-6 kg  num_ports=foundation.enum.numPorts2.one  m_specify=off  m_priority=High  m=1 kg  m_nominal_specify=off  m_nominal_value=1  m_nominal_unit=kg  T_specify=on  T_priority=Low  T=293.15 K  T_nominal_specify=off  T_nominal_value=1  T_nominal_unit=K  Q_specify=off  Q_priority=None  Q=0 W  Q_nominal_specify=off  Q_nominal_value=1  Q_nominal_unit=W
  Voltage Sensor : fl_lib/Electrical/Electrical Sensors/Voltage Sensor
  docking charger : simulink/Sources/Waveform Generator  OutMin=[]  OutMax=[]  OutDataTypeStr=double  SelectedSignal=1  Signals=step(5.5, 10000, 2.88)  BlockNames=MultiportSwitch_f5c123cea90d475  SampleTime=0.1
  1 : PMIOPort  Side=Left
  D : Outport
  S3C : Outport  Port=2
  S3V : Outport  Port=3
  wires:
  " 11"/1 -> [CL]
  " 4"/1 -> [Ch]
  docking charger/1 -> Simulink-PS Converter7/1
  [Ch] -> Power of Dock/1  "Charger"
  [CL] -> Power of Dock/2  "Clamps"
  PS-Simulink Converter/1 -> D/1
  PS-Simulink Converter1/1 -> S3C/1
  PS-Simulink Converter2/1 -> S3V/1
  connections:
  Inductor2/RConn1 -- Resistor4/LConn1
  Charger/LConn2 -- Power Sensor8/LConn2
  " 4"/LConn1 -- Power Sensor8/RConn1
  Charger/RConn1 -- Power Sensor8/LConn3 -- Voltage Sensor/RConn2 -- Electrical Reference2/LConn1 -- Power Sensor1/LConn3 -- Resistor4/RConn1 -- Resistor3/RConn1 -- Power Sensor/LConn3 -- Resistor2/RConn1
  " 11"/LConn1 -- Power Sensor/RConn1
  Simulink-PS Converter7/RConn1 -- Charger/LConn1
  Thermal Mass4/LConn1 -- Charger/LConn3
  Inductor1/RConn1 -- Resistor3/LConn1
  Power Sensor8/LConn1 -- Power Sensor1/LConn2 -- Power Sensor/LConn1
  Inductor1/LConn1 -- Inductor2/LConn1 -- Inductor/LConn1 -- Power Sensor/LConn2
  Inductor/RConn1 -- Resistor2/LConn1
  PS-Simulink Converter/LConn1 -- Power Sensor1/RConn1
  Current Sensor/RConn2 -- Power Sensor1/LConn1
  Current Sensor/LConn1 -- Voltage Sensor/LConn1 -- 1/RConn1
  PS-Simulink Converter1/LConn1 -- Current Sensor/RConn1
  PS-Simulink Converter2/LConn1 -- Voltage Sensor/RConn1

== matlab function IDP2_Shehab_Electrical_Systems_Model/MATLAB Function ==
  data: S3 output; fault input; S2 output; initialmode input; mode output
function [S3, S2, mode] = controller(fault, initialmode)

S2 = double(1);
S3 = double(0);
mode = double(1);

if fault == 1
    mode = double(3);
    S2 = double(0);
    S3 = double(0);

elseif initialmode == 2
    mode = double(2);
    S2 = double(1);
    S3 = double(1);

else
    mode = double(1);
    S2 = double(1);
    S3 = double(0);
end

== matlab function IDP2_Shehab_Electrical_Systems_Model/MATLAB Function2 ==
  data: B1V input; B1C input; B2V input; B2C input; fault output; fault_location output; B3V input; IM input
function [fault, fault_location] = protection(B1V, B1C, B2V, B2C,B3V,IM)

fault = double(0);
fault_location = double(0);


if B1V < 21 || B1C <2
    % Emergency at Branch 1 
    fault = double(1);
    fault_location = double(1);
    
elseif B2V < 21 || B2C <1
    % Emergency at Branch 2
    fault = double(1);
    fault_location = double(2);

elseif IM == 2 && (B3V < 20 )
    % Emergency at Branch 3 
    fault = double(1);
    fault_location = double(3);

else
    fault = double(0);
    fault_location = double(0);
end
